simulink model "CoETS_NTC"  (R2016b)
settings: configuration reference "CodeGenConfigSet" (kept outside this file)
values from neighbouring files (symbols this model uses):
  CoETS_trqNTCInrAct_C = Calibration.Parameter    [init_CoETS_NTC.m]
  CoETS_trqNTCInrMax_C = Calibration.Parameter    [init_CoETS_NTC.m]
  CoETS_trqNTCLim_C = Calibration.Parameter    [init_CoETS_NTC.m]
settings Model: Creator=lenovo  LastModifiedBy=lenovo
settings ConfigSetRef: SourceLocation=Base Workspace

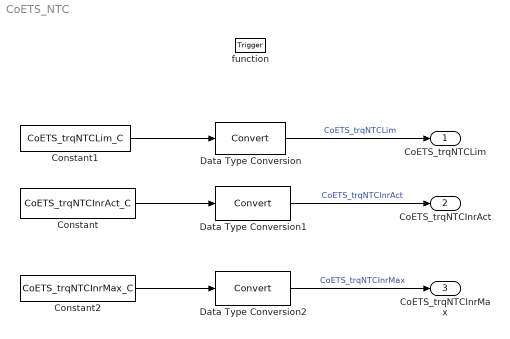
== system CoETS_NTC ==
  function : TriggerPort  TriggerType=function-call  VariantControl=Variant
  Constant : Constant  Value=CoETS_trqNTCInrAct_C
  Constant1 : Constant  Value=CoETS_trqNTCLim_C
  Constant2 : Constant  Value=CoETS_trqNTCInrMax_C
  Data Type Conversion : DataTypeConversion
  Data Type Conversion1 : DataTypeConversion
  Data Type Conversion2 : DataTypeConversion
  CoETS_trqNTCLim : Outport  Tag=Nm  Description=NTC torque limitation (0 in braking, ramped to max in braked to fired  OutMin=0  OutMax=1000  OutDataTypeStr=Trq_Nm
  CoETS_trqNTCInrAct : Outport  Tag=Nm  Description=Actual braking torque  Port=2  OutMin=-3276.8  OutMax=3276.7  OutDataTypeStr=Trq_Nm
  CoETS_trqNTCInrMax : Outport  Tag=Nm  Description=Maximum available braking torque  Port=3  OutMin=-3276.8  OutMax=3276.7  OutDataTypeStr=Trq_Nm
  wires:
  Constant1/1 -> Data Type Conversion/1
  Data Type Conversion/1 -> CoETS_trqNTCLim/1  "CoETS_trqNTCLim"
  Constant/1 -> Data Type Conversion1/1
  Data Type Conversion1/1 -> CoETS_trqNTCInrAct/1  "CoETS_trqNTCInrAct"
  Constant2/1 -> Data Type Conversion2/1
  Data Type Conversion2/1 -> CoETS_trqNTCInrMax/1  "CoETS_trqNTCInrMax"
